simulink model "mrac_lyap"  (R2021b)
settings: Solver=FixedStepAuto  StartTime=0.0  StopTime=600  FixedStep=1  RelTol=1e-3
undefined symbols (not defined in the file or in its folder): setSimFunc
settings Model: Creator=ismt  LastModifiedBy=ismt

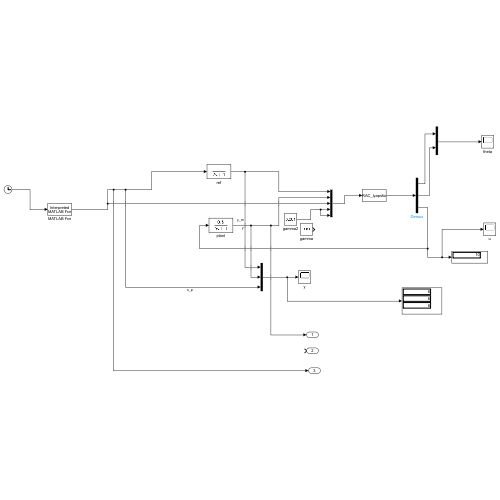
[thumbnail: Simulink's stored preview of the top-level diagram]
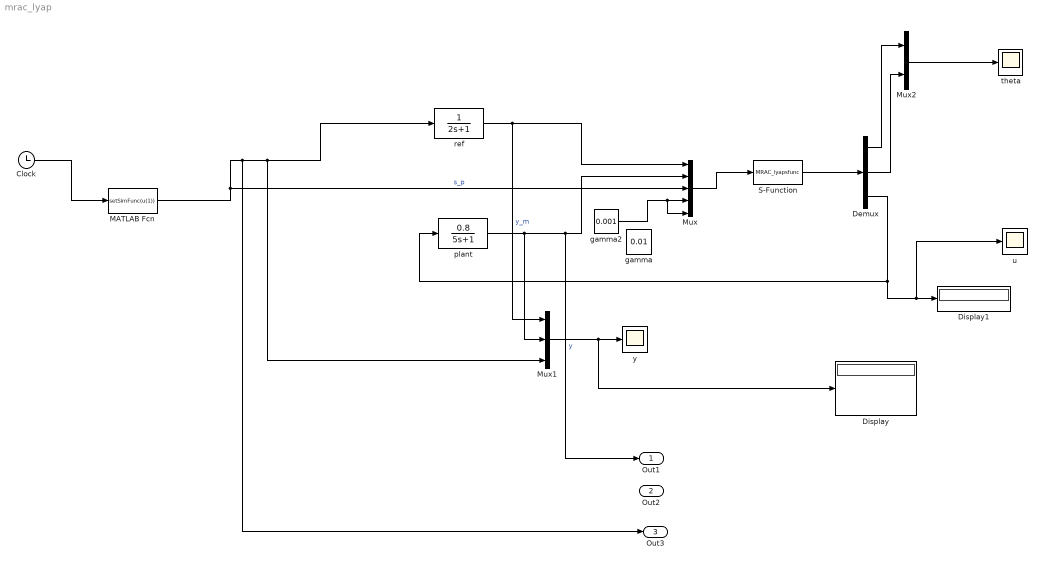
== system mrac_lyap ==
  Clock : Clock
  Demux : Demux  Outputs=3
  Display : Display
  Display1 : Display
  MATLAB Fcn : MATLABFcn  MATLABFcn=setSimFunc(u(1))
  Mux : Mux  Inputs=5
  Mux1 : Mux  Inputs=3
  Mux2 : Mux  Inputs=2
  S-Function : S-Function  FunctionName=MRAC_lyapsfunc  SFunctionDeploymentMode=off  EnableBusSupport=off
  gamma : Constant  Value=0.01
  gamma2 : Constant  Value=0.001
  plant : TransferFcn  Numerator=[0.8]  Denominator=[5 1]
  ref : TransferFcn  Denominator=[2 1]
  theta : Scope
  u : Scope
  y : Scope
  Out1 : Outport
  Out2 : Outport  Port=2
  Out3 : Outport  Port=3
  wires:
  Clock/1 -> MATLAB Fcn/1
  Mux/1 -> S-Function/1
  Mux1/1 -> Display/1, y/1
  ref/1 -> Mux/1, Mux1/1  "y_m"
  MATLAB Fcn/1 -> ref/1, Mux1/3, Out3/1, Mux/3  "s_p"
  plant/1 -> Mux1/2, Mux/2, Out1/1  "y"
  gamma2/1 -> Mux/5, Mux/4
  S-Function/1 -> Demux/1
  Mux2/1 -> theta/1
  Demux/1 -> Mux2/1
  Demux/2 -> Mux2/2
  Demux/3 -> u/1, Display1/1, plant/1
